simulink model "ctrl_custom"  (R2016b)
settings: Solver=ode4  StartTime=0.0  StopTime=inf  FixedStep=0.01  RelTol=1e-3  EnableMultiTasking=on
undefined symbols (not defined in the file): alpha1, alpha2, C1, C2, D, inv_M, L_1, L_2, L_3
libraries: lib x7, simulink x3, simulink_extras x1
(part 2 of 2)

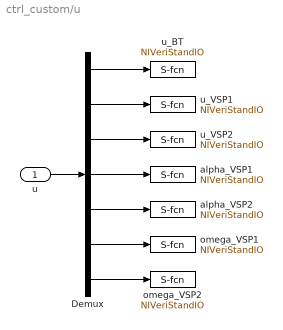
== system ctrl_custom/u ==
  u : Inport
  Demux : Demux  Outputs=7
  alpha_VSP1 : S-Function  Priority=4  FunctionName=NIVeriStandIO  Parameters=width dtype portnum stime stype btype  SFunctionDeploymentMode=off  EnableBusSupport=off  mask(NI VeriStand Outport){portnum=4, width=-1, stime=-1, dtype=auto, stype=auto, btype=0}
      mask prompts: portnum "Port number:"; width "Port dimensions (-1 for dynamically sized):"; stime "Sample time (-1 for inherited):"; dtype "Data type:"; stype "Signal type:"; btype "Block type:"
      mask help: Use this outport on any level of nested subsystems to allow NI VeriStand software to map signals to it.
      mask init:
      | NIVeriStandIO_init;
      settings: CopyFcn=NIVeriStand_MDL_functions('', 'IO_copy');  DeleteFcn=NIVeriStand_MDL_functions('', 'IO_delete');  MoveFcn=set_param(gcb, 'Mask', 'on');
      mask Callback portnum: NIVeriStand_MDL_functions('', 'IO_setportnum');
      mask TypeOptions dtype: auto | double | single | int8 | uint8 | int16 | uint16 | int32 | uint32 | boolean
      mask Callback dtype: NIVeriStand_MDL_functions('', 'IO_booleansignal');
      mask TypeOptions stype: auto | real | complex
      mask Display:
      | patch([-x x], [-y y], [.90980 .81960 .32156]);
      | plot([xrad -x x xrad], [yrad -y y yrad]);
      | fprintf('NI Out%d', portnum);
  alpha_VSP2 : S-Function  Priority=1  FunctionName=NIVeriStandIO  Parameters=width dtype portnum stime stype btype  SFunctionDeploymentMode=off  EnableBusSupport=off  mask(NI VeriStand Outport){portnum=1, width=-1, stime=-1, dtype=auto, stype=auto, btype=0}
      mask prompts: portnum "Port number:"; width "Port dimensions (-1 for dynamically sized):"; stime "Sample time (-1 for inherited):"; dtype "Data type:"; stype "Signal type:"; btype "Block type:"
      mask help: Use this outport on any level of nested subsystems to allow NI VeriStand software to map signals to it.
      mask init:
      | NIVeriStandIO_init;
      settings: CopyFcn=NIVeriStand_MDL_functions('', 'IO_copy');  DeleteFcn=NIVeriStand_MDL_functions('', 'IO_delete');  MoveFcn=set_param(gcb, 'Mask', 'on');
      mask Callback portnum: NIVeriStand_MDL_functions('', 'IO_setportnum');
      mask TypeOptions dtype: auto | double | single | int8 | uint8 | int16 | uint16 | int32 | uint32 | boolean
      mask Callback dtype: NIVeriStand_MDL_functions('', 'IO_booleansignal');
      mask TypeOptions stype: auto | real | complex
      mask Display:
      | patch([-x x], [-y y], [.90980 .81960 .32156]);
      | plot([xrad -x x xrad], [yrad -y y yrad]);
      | fprintf('NI Out%d', portnum);
  omega_VSP1 : S-Function  Priority=2  FunctionName=NIVeriStandIO  Parameters=width dtype portnum stime stype btype  SFunctionDeploymentMode=off  EnableBusSupport=off  mask(NI VeriStand Outport){portnum=2, width=-1, stime=-1, dtype=auto, stype=auto, btype=0}
      mask prompts: portnum "Port number:"; width "Port dimensions (-1 for dynamically sized):"; stime "Sample time (-1 for inherited):"; dtype "Data type:"; stype "Signal type:"; btype "Block type:"
      mask help: Use this outport on any level of nested subsystems to allow NI VeriStand software to map signals to it.
      mask init:
      | NIVeriStandIO_init;
      settings: CopyFcn=NIVeriStand_MDL_functions('', 'IO_copy');  DeleteFcn=NIVeriStand_MDL_functions('', 'IO_delete');  MoveFcn=set_param(gcb, 'Mask', 'on');
      mask Callback portnum: NIVeriStand_MDL_functions('', 'IO_setportnum');
      mask TypeOptions dtype: auto | double | single | int8 | uint8 | int16 | uint16 | int32 | uint32 | boolean
      mask Callback dtype: NIVeriStand_MDL_functions('', 'IO_booleansignal');
      mask TypeOptions stype: auto | real | complex
      mask Display:
      | patch([-x x], [-y y], [.90980 .81960 .32156]);
      | plot([xrad -x x xrad], [yrad -y y yrad]);
      | fprintf('NI Out%d', portnum);
  omega_VSP2 : S-Function  Priority=3  FunctionName=NIVeriStandIO  Parameters=width dtype portnum stime stype btype  SFunctionDeploymentMode=off  EnableBusSupport=off  mask(NI VeriStand Outport){portnum=3, width=-1, stime=-1, dtype=auto, stype=auto, btype=0}
      mask prompts: portnum "Port number:"; width "Port dimensions (-1 for dynamically sized):"; stime "Sample time (-1 for inherited):"; dtype "Data type:"; stype "Signal type:"; btype "Block type:"
      mask help: Use this outport on any level of nested subsystems to allow NI VeriStand software to map signals to it.
      mask init:
      | NIVeriStandIO_init;
      settings: CopyFcn=NIVeriStand_MDL_functions('', 'IO_copy');  DeleteFcn=NIVeriStand_MDL_functions('', 'IO_delete');  MoveFcn=set_param(gcb, 'Mask', 'on');
      mask Callback portnum: NIVeriStand_MDL_functions('', 'IO_setportnum');
      mask TypeOptions dtype: auto | double | single | int8 | uint8 | int16 | uint16 | int32 | uint32 | boolean
      mask Callback dtype: NIVeriStand_MDL_functions('', 'IO_booleansignal');
      mask TypeOptions stype: auto | real | complex
      mask Display:
      | patch([-x x], [-y y], [.90980 .81960 .32156]);
      | plot([xrad -x x xrad], [yrad -y y yrad]);
      | fprintf('NI Out%d', portnum);
  u_BT : S-Function  Priority=5  FunctionName=NIVeriStandIO  Parameters=width dtype portnum stime stype btype  SFunctionDeploymentMode=off  EnableBusSupport=off  mask(NI VeriStand Outport){portnum=5, width=-1, stime=-1, dtype=auto, stype=auto, btype=0}
      mask prompts: portnum "Port number:"; width "Port dimensions (-1 for dynamically sized):"; stime "Sample time (-1 for inherited):"; dtype "Data type:"; stype "Signal type:"; btype "Block type:"
      mask help: Use this outport on any level of nested subsystems to allow NI VeriStand software to map signals to it.
      mask init:
      | NIVeriStandIO_init;
      settings: CopyFcn=NIVeriStand_MDL_functions('', 'IO_copy');  DeleteFcn=NIVeriStand_MDL_functions('', 'IO_delete');  MoveFcn=set_param(gcb, 'Mask', 'on');
      mask Callback portnum: NIVeriStand_MDL_functions('', 'IO_setportnum');
      mask TypeOptions dtype: auto | double | single | int8 | uint8 | int16 | uint16 | int32 | uint32 | boolean
      mask Callback dtype: NIVeriStand_MDL_functions('', 'IO_booleansignal');
      mask TypeOptions stype: auto | real | complex
      mask Display:
      | patch([-x x], [-y y], [.90980 .81960 .32156]);
      | plot([xrad -x x xrad], [yrad -y y yrad]);
      | fprintf('NI Out%d', portnum);
  u_VSP1 : S-Function  Priority=6  FunctionName=NIVeriStandIO  Parameters=width dtype portnum stime stype btype  SFunctionDeploymentMode=off  EnableBusSupport=off  mask(NI VeriStand Outport){portnum=6, width=-1, stime=-1, dtype=auto, stype=auto, btype=0}
      mask prompts: portnum "Port number:"; width "Port dimensions (-1 for dynamically sized):"; stime "Sample time (-1 for inherited):"; dtype "Data type:"; stype "Signal type:"; btype "Block type:"
      mask help: Use this outport on any level of nested subsystems to allow NI VeriStand software to map signals to it.
      mask init:
      | NIVeriStandIO_init;
      settings: CopyFcn=NIVeriStand_MDL_functions('', 'IO_copy');  DeleteFcn=NIVeriStand_MDL_functions('', 'IO_delete');  MoveFcn=set_param(gcb, 'Mask', 'on');
      mask Callback portnum: NIVeriStand_MDL_functions('', 'IO_setportnum');
      mask TypeOptions dtype: auto | double | single | int8 | uint8 | int16 | uint16 | int32 | uint32 | boolean
      mask Callback dtype: NIVeriStand_MDL_functions('', 'IO_booleansignal');
      mask TypeOptions stype: auto | real | complex
      mask Display:
      | patch([-x x], [-y y], [.90980 .81960 .32156]);
      | plot([xrad -x x xrad], [yrad -y y yrad]);
      | fprintf('NI Out%d', portnum);
  u_VSP2 : S-Function  Priority=7  FunctionName=NIVeriStandIO  Parameters=width dtype portnum stime stype btype  SFunctionDeploymentMode=off  EnableBusSupport=off  mask(NI VeriStand Outport){portnum=7, width=-1, stime=-1, dtype=auto, stype=auto, btype=0}
      mask prompts: portnum "Port number:"; width "Port dimensions (-1 for dynamically sized):"; stime "Sample time (-1 for inherited):"; dtype "Data type:"; stype "Signal type:"; btype "Block type:"
      mask help: Use this outport on any level of nested subsystems to allow NI VeriStand software to map signals to it.
      mask init:
      | NIVeriStandIO_init;
      settings: CopyFcn=NIVeriStand_MDL_functions('', 'IO_copy');  DeleteFcn=NIVeriStand_MDL_functions('', 'IO_delete');  MoveFcn=set_param(gcb, 'Mask', 'on');
      mask Callback portnum: NIVeriStand_MDL_functions('', 'IO_setportnum');
      mask TypeOptions dtype: auto | double | single | int8 | uint8 | int16 | uint16 | int32 | uint32 | boolean
      mask Callback dtype: NIVeriStand_MDL_functions('', 'IO_booleansignal');
      mask TypeOptions stype: auto | real | complex
      mask Display:
      | patch([-x x], [-y y], [.90980 .81960 .32156]);
      | plot([xrad -x x xrad], [yrad -y y yrad]);
      | fprintf('NI Out%d', portnum);
  wires:
  u/1 -> Demux/1
  Demux/1 -> u_BT/1
  Demux/2 -> u_VSP1/1
  Demux/3 -> u_VSP2/1
  Demux/4 -> alpha_VSP1/1
  Demux/5 -> alpha_VSP2/1
  Demux/6 -> omega_VSP1/1
  Demux/7 -> omega_VSP2/1

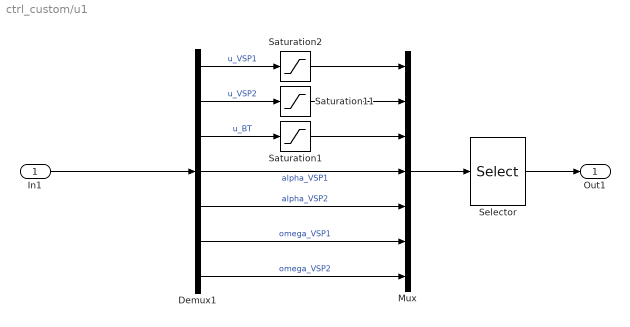
== system ctrl_custom/u1 ==
  In1 : Inport
  Demux1 : Demux  Outputs=7
  Mux : Mux  Inputs=7
  Saturation1 : Saturate  UpperLimit=1  LowerLimit=-1
  Saturation11 : Saturate  UpperLimit=1  LowerLimit=0
  Saturation2 : Saturate  UpperLimit=1  LowerLimit=0
  Selector : Selector  InputPortWidth=7  IndexOptions=Index vector (dialog)  Indices=[3 1 2 4 5 6 7]  OutputSizes=1
  Out1 : Outport
  wires:
  In1/1 -> Demux1/1
  Demux1/1 -> Saturation2/1  "u_VSP1"
  Demux1/2 -> Saturation11/1  "u_VSP2"
  Demux1/3 -> Saturation1/1  "u_BT"
  Demux1/4 -> Mux/4  "alpha_VSP1"
  Demux1/5 -> Mux/5  "alpha_VSP2"
  Demux1/6 -> Mux/6  "omega_VSP1"
  Demux1/7 -> Mux/7  "omega_VSP2"
  Mux/1 -> Selector/1
  Saturation11/1 -> Mux/2
  Saturation1/1 -> Mux/3
  Saturation2/1 -> Mux/1
  Selector/1 -> Out1/1

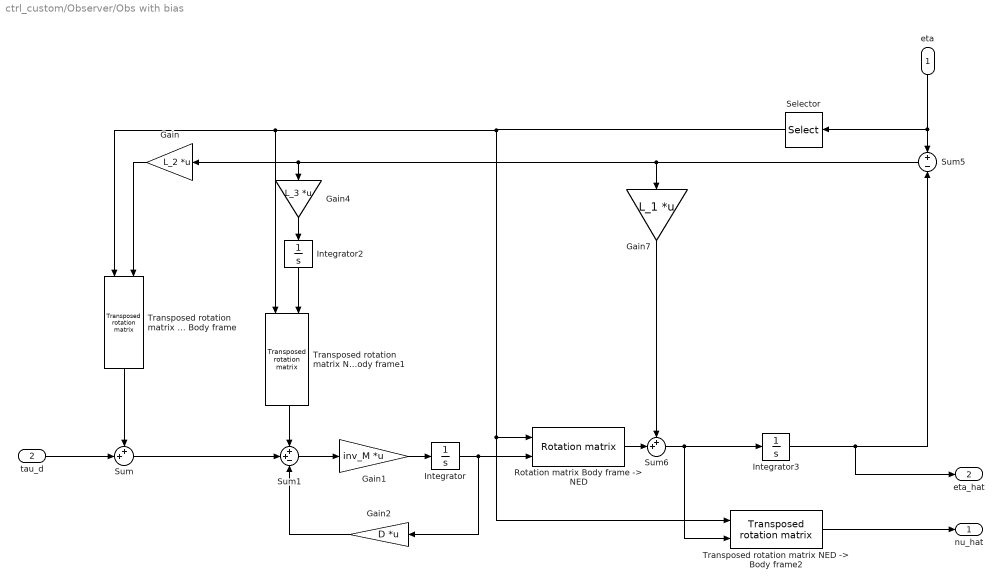
== system ctrl_custom/Observer/Obs with bias ==
  eta : Inport
  tau_d : Inport  Port=2
  Gain : Gain  Gain=L_2  Multiplication=Matrix(K*u)
  Gain1 : Gain  Gain=inv_M  Multiplication=Matrix(K*u)
  Gain2 : Gain  Gain=D  Multiplication=Matrix(K*u)
  Gain4 : Gain  Gain=L_3  Multiplication=Matrix(K*u)
  Gain7 : Gain  Gain=L_1  Multiplication=Matrix(K*u)
  Integrator : Integrator
  Integrator2 : Integrator
  Integrator3 : Integrator
  "Rotation matrix Body frame -> NED" : lib/Rotation matrix
  Selector : Selector  InputPortWidth=3  IndexOptions=Index vector (dialog)  Indices=[ 3]  OutputSizes=1
  Sum : Sum  Inputs=++|
  Sum1 : Sum  Inputs=++-
  Sum5 : Sum  Inputs=+|-
  Sum6 : Sum  Inputs=++|
  "Transposed rotation matrix NED -> Body frame" : lib/Transposed rotation matrix
  "Transposed rotation matrix NED -> Body frame1" : lib/Transposed rotation matrix
  "Transposed rotation matrix NED -> Body frame2" : lib/Transposed rotation matrix
  nu_hat : Outport
  eta_hat : Outport  Port=2
  wires:
  tau_d/1 -> Sum/2
  Gain/1 -> "Transposed rotation matrix NED -> Body frame"/2
  "Transposed rotation matrix NED -> Body frame"/1 -> Sum/1
  "Transposed rotation matrix NED -> Body frame1"/1 -> Sum1/1
  Gain1/1 -> Integrator/1
  Integrator/1 -> Gain2/1, "Rotation matrix Body frame -> NED"/2
  "Rotation matrix Body frame -> NED"/1 -> Sum6/2
  Sum6/1 -> "Transposed rotation matrix NED -> Body frame2"/2, Integrator3/1
  Gain2/1 -> Sum1/3
  Sum/1 -> Sum1/2
  Integrator2/1 -> "Transposed rotation matrix NED -> Body frame1"/2
  Gain4/1 -> Integrator2/1
  Gain7/1 -> Sum6/1
  Sum1/1 -> Gain1/1
  eta/1 -> Selector/1, Sum5/1
  "Transposed rotation matrix NED -> Body frame2"/1 -> nu_hat/1
  Integrator3/1 -> Sum5/2, eta_hat/1
  Sum5/1 -> Gain4/1, Gain/1, Gain7/1
  Selector/1 -> "Transposed rotation matrix NED -> Body frame2"/1, "Rotation matrix Body frame -> NED"/1, "Transposed rotation matrix NED -> Body frame"/1, "Transposed rotation matrix NED -> Body frame1"/1

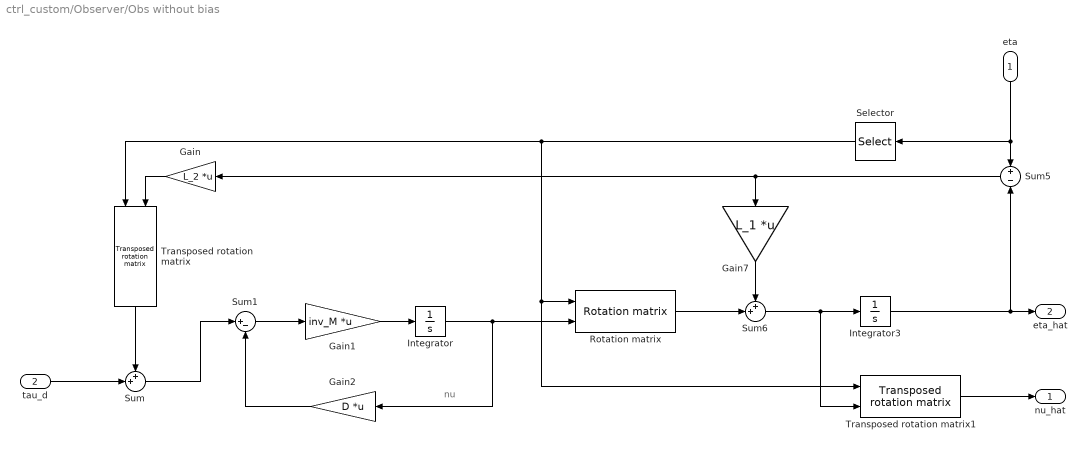
== system ctrl_custom/Observer/Obs without bias ==
  note: nu
  eta : Inport
  tau_d : Inport  Port=2
  Gain : Gain  Gain=L_2  Multiplication=Matrix(K*u)
  Gain1 : Gain  Gain=inv_M  Multiplication=Matrix(K*u)
  Gain2 : Gain  Gain=D  Multiplication=Matrix(K*u)
  Gain7 : Gain  Gain=L_1  Multiplication=Matrix(K*u)
  Integrator : Integrator
  Integrator3 : Integrator
  Rotation matrix : lib/Rotation matrix
  Selector : Selector  InputPortWidth=3  IndexOptions=Index vector (dialog)  Indices=[ 3]  OutputSizes=1
  Sum : Sum  Inputs=++|
  Sum1 : Sum  Inputs=|+-
  Sum5 : Sum  Inputs=+|-
  Sum6 : Sum  Inputs=++|
  Transposed rotation matrix : lib/Transposed rotation matrix
  Transposed rotation matrix1 : lib/Transposed rotation matrix
  nu_hat : Outport
  eta_hat : Outport  Port=2
  wires:
  Sum/1 -> Sum1/1
  Sum6/1 -> Transposed rotation matrix1/2, Integrator3/1
  Transposed rotation matrix1/1 -> nu_hat/1
  Gain7/1 -> Sum6/1
  Rotation matrix/1 -> Sum6/2
  Sum5/1 -> Gain/1, Gain7/1
  Gain1/1 -> Integrator/1
  tau_d/1 -> Sum/2
  Integrator3/1 -> Sum5/2, eta_hat/1
  Gain/1 -> Transposed rotation matrix/2
  Transposed rotation matrix/1 -> Sum/1
  Sum1/1 -> Gain1/1
  eta/1 -> Selector/1, Sum5/1
  Selector/1 -> Transposed rotation matrix/1, Transposed rotation matrix1/1, Rotation matrix/1
  Gain2/1 -> Sum1/2
  Integrator/1 -> Gain2/1, Rotation matrix/2

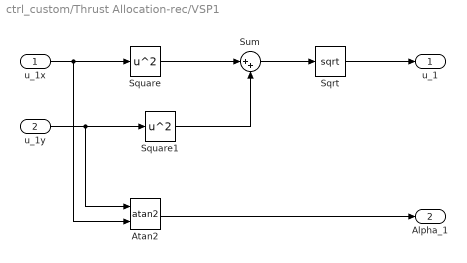
== system ctrl_custom/Thrust Allocation-rec/VSP1 ==
  u_1x : Inport
  u_1y : Inport  Port=2
  Atan2 : Trigonometry  Operator=atan2
  Sqrt : Sqrt  SaturateOnIntegerOverflow=on
  Square : Math  Operator=square  SaturateOnIntegerOverflow=on
  Square1 : Math  Operator=square  SaturateOnIntegerOverflow=on
  Sum : Sum  Inputs=|++
  u_1 : Outport
  Alpha_1 : Outport  Port=2
  wires:
  u_1x/1 -> Atan2/2, Square/1
  u_1y/1 -> Atan2/1, Square1/1
  Square/1 -> Sum/1
  Square1/1 -> Sum/2
  Sum/1 -> Sqrt/1
  Sqrt/1 -> u_1/1
  Atan2/1 -> Alpha_1/1

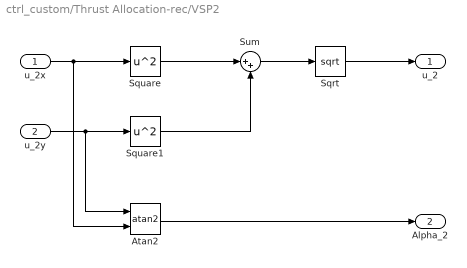
== system ctrl_custom/Thrust Allocation-rec/VSP2 ==
  u_2x : Inport
  u_2y : Inport  Port=2
  Atan2 : Trigonometry  Operator=atan2
  Sqrt : Sqrt  SaturateOnIntegerOverflow=on
  Square : Math  Operator=square  SaturateOnIntegerOverflow=on
  Square1 : Math  Operator=square  SaturateOnIntegerOverflow=on
  Sum : Sum  Inputs=|++
  u_2 : Outport
  Alpha_2 : Outport  Port=2
  wires:
  Square/1 -> Sum/1
  Square1/1 -> Sum/2
  Sum/1 -> Sqrt/1
  Sqrt/1 -> u_2/1
  u_2x/1 -> Atan2/2, Square/1
  Atan2/1 -> Alpha_2/1
  u_2y/1 -> Atan2/1, Square1/1

== matlab function ctrl_custom/MATLAB Function1 ==
  data: x output; u input; y output
function [x,y] = fcn(u)

x = 1;
y = 0;
if u == 1
    x = 1;
    y = 0;
end

if u == 2
    x = 0;
    y = 1;
end

== matlab function ctrl_custom/Switch_function1 ==
  data: ArrowL input; switch_signal output; ArrowR input; temp input
%% Function that takes in impulse button sigals [0,1] and sends out a 
% different signal depentent pn which button has been pressed

function switch_signal = fcn(ArrowL,ArrowR,temp)
%#codegen
persistent signal;

signal = temp;

if ArrowL ~= 0
    signal = 1;
end

if ArrowR ~= 0
    signal = 2;
end


switch_signal = signal;
